simulink model "ArmStateMachineModel"  (Simulink 6.2)
settings: Solver=ode45  SolverMode=SingleTasking  StartTime=0.0  StopTime=10.0  RelTol=1e-3  AbsTol=1e-6
settings Model: Creator=The MathWorks Inc.  LastModifiedBy=suarezjl  ExtModeTrigMode=oneshot  ExtModeArmWhenConnect=off  ExtModeAutoUpdateStatusClock=off
settings DataIOCC: LimitDataPoints=off  SignalLoggingName=logsOut
settings OptimizationCC: BooleanDataType=off  InlineInvariantSignals=on
settings DebuggingCC: CheckExecutionContextPreStartOutputMsg=on  CheckExecutionContextRuntimeOutputMsg=on  IntegerOverflowMsg=none
settings HardwareCC: TargetUnknown=on
settings ModelReferenceCC: UpdateModelReferenceTargets=IfOutOfDate

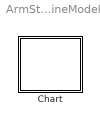
== system ArmStateMachineModel ==
  Chart : Stateflow chart

== stateflow chart Chart ==
  state Initialize
    Popeye\RightArmAgent\SampleIndPressures\Disable_ZMasking()
    Popeye\RightArmAgent\HomingController\ComputeHomingPressures()
    Popeye\RightArmAgent\SampleIndPressures\HW_IO_6()
  state MoveArm
    Popeye\RightArmAgent\SampleIndPressures\Enable_ZMasking()
    Popeye\RightArmAgent\SampleIndPressures\WriteHomeAngles()
    Popeye\RightArmAgent\SampleIndPressures\HW_IO_6()
    Popeye\RightArmAgent\PIDNonLinCtrl\PID_NonLin_6Press()
  state ComputeInitialCartesianPositions
    Popeye\RightArmAgent\ForwardKinematics\ForwardKinematics()
    Popeye\RightArmAgent\InverseKinematics\InverseKinematics()
  state PID_NonLinCtrlLoop
    Popeye\RightArmAgent\PIDNonLinCtrl\PID_NonLin_12Press()
    Popeye\RightArmAgent\SampleIndPressures\HW_IO_12()
    Popeye\RightArmAgent\PIDNonLinCtrl\Read_CurrentPressure()
    Popeye\RightArmAgent\ForwardKinematics\ForwardKinematics()
    Popeye\RightArmAgent\InverseKinematics\InverseKinematics()
    Popeye\RightArmAgent\Filter\FilterDesiredAngles()
  state Stop
    Popeye\RightArmAgent\StateMahcine.Stop()
  Initialize -> MoveArm : Signal="Homer"
  MoveArm -> ComputeInitialCartesianPositions : Signal="Sampler"
  ComputeInitialCartesianPositions -> PID_NonLinCtrlLoop : Always
  (default) -> PID_NonLinCtrlLoop [order 2] : Always
  (default) -> Initialize [order 1] : Start
  PID_NonLinCtrlLoop -> Stop : Signal="Stop"
